simulink model "Fullmodelcontrol"  (R2020a)
settings: Solver=VariableStepAuto  StartTime=0.0  StopTime=10.0  RelTol=1e-3
values from neighbouring files (symbols this model uses):
  Ar = pi*D*D/4    (= 0.00465662571078)    [parameters.m]
  Cd = 0.23    [parameters.m]
  d = 0.081    [parameters.m]
  g = 9.81    [parameters.m]
  Ixx = 2.156e-3    (= 0.002156)    [parameters.m]
  l = 0.32    [parameters.m]
  m = 276.72e-3    (= 0.27672)    [parameters.m]
  rho = 1.225    [parameters.m]
  Thrust_timeC6 = (thrustprofileC6(:,1))'    [parameters.m]
  ThrustNtC6 = (thrustprofileC6(:,2))'    [parameters.m]
libraries: simulink x4, vrlib x2, dspsrcs4 x1
settings Model: Creator=sahil  LastModifiedBy=sahil

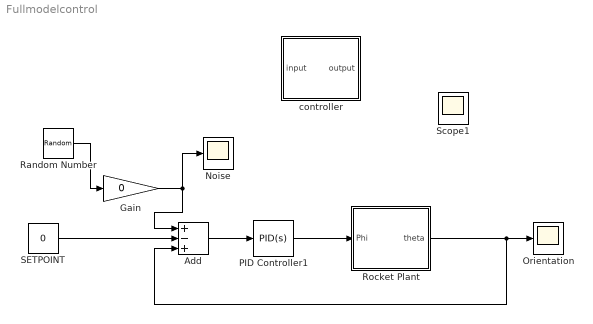
== system Fullmodelcontrol ==
  Add : Sum  Inputs=+-+
  Gain : Gain  Gain=0
  Noise : Scope
  Orientation : Scope
  PID Controller1 : simulink/Continuous/PID Controller  Controller=PID  Form=Parallel  TimeDomain=Continuous-time  UseExternalTs=off  SampleTime=-1  IntegratorMethod=Forward Euler  FilterMethod=Forward Euler  ControllerParametersSource=internal  P=0.142515145482664  I=0.0728938771028704  D=0.0532267076951464  UseFilter=on  N=36.46824066771  TunerSelectOption=Transfer Function Based (PID Tuner App)  InitialConditionSource=internal  InitialConditionForIntegrator=0  InitialConditionForFilter=0  DifferentiatorICPrevScaledInput=0  ExternalReset=none  TrackingMode=off  Kt=1  LimitOutput=on  UpperSaturationLimit=0.087  LowerSaturationLimit=-0.087  LinearizeAsGain=off  AntiWindupMode=none  Kb=1  POutMin=[]  POutMax=[]  IOutMin=[]  IOutMax=[]  DOutMin=[]  DOutMax=[]  NOutMin=[]  NOutMax=[]  SumOutMin=[]  SumOutMax=[]  SaturationOutMin=[]  SaturationOutMax=[]  PParamMin=[]  PParamMax=[]  IParamMin=[]  IParamMax=[]  DParamMin=[]  DParamMax=[]  NParamMin=[]  NParamMax=[]  KbParamMin=[]  KbParamMax=[]  KtParamMin=[]  KtParamMax=[]  KbOutMin=[]  KbOutMax=[]  KtOutMin=[]  KtOutMax=[]  IntegratorOutMin=[]  IntegratorOutMax=[]  FilterOutMin=[]  FilterOutMax=[]  SumI1OutMin=[]  SumI1OutMax=[]  SumI2OutMin=[]  SumI2OutMax=[]  SumI3OutMin=[]  SumI3OutMax=[]  SumI4OutMin=[]  SumI4OutMax=[]  SumDOutMin=[]  SumDOutMax=[]  DifferentiatorOutMin=[]  DifferentiatorOutMax=[]  FilterDiffOutCoefMin=[]  FilterDiffOutCoefMax=[]  ReciprocalOutMin=[]  ReciprocalOutMax=[]  SumDenOutMin=[]  SumDenOutMax=[]  SumNumOutMin=[]  SumNumOutMax=[]  DivideOutMin=[]  DivideOutMax=[]  UdiffTsProdOutMin=[]  UdiffTsProdOutMax=[]  NTsProdOutMin=[]  NTsProdOutMax=[]  UintegralTsProdOutMin=[]  UintegralTsProdOutMax=[]  UngainTsProdOutMin=[]  UngainTsProdOutMax=[]  IntegratorContinuousStateAttributes=''  IntegratorStateMustResolveToSignalObject=off  IntegratorRTWStateStorageClass=Auto  FilterContinuousStateAttributes=''  FilterStateMustResolveToSignalObject=off  FilterRTWStateStorageClass=Auto  ParallelPVariant=InternalParameters  IdealPVariant=Disabled  IVariant=InternalParameters  DVariant=InternalParameters  IntegratorVariant=Continuous  SatVariant=Enabled  AWVariant=Passthrough  PCopyVariant=Disabled  TRVariant=Disabled  FdbkBlocksVariant=Forward  IdealPFdbkVariant=Disabled  SatFdbkVariant=Disabled  DerivativeFilterVariant=ContFilter  NVariant=InternalParameters  NCopyVariant=Disabled  FilterICVariant=InternalICsFilter  IntegratorICVariant=InternalICs  ExternalResetVariant=Disabled  TRSumVariant=Passthrough  SumFdbkVariant=Disabled  SumVariant=Sum_PID  TsampFilterVariant=InternalTs  TsampNgainVariant=Passthrough  TsampIntegralVariant=Passthrough
  Random Number : RandomNumber  SampleTime=0.1
  Rocket Plant : Subsystem
  SETPOINT : Constant  Value=0
  Scope1 : Scope
  controller : Subsystem
  wires:
  Rocket Plant/1(theta) -> Add/3, Orientation/1
  PID Controller1/1 -> Rocket Plant/1(Phi)
  Random Number/1 -> Gain/1
  Gain/1 -> Add/1, Noise/1
  SETPOINT/1 -> Add/2
  Add/1 -> PID Controller1/1

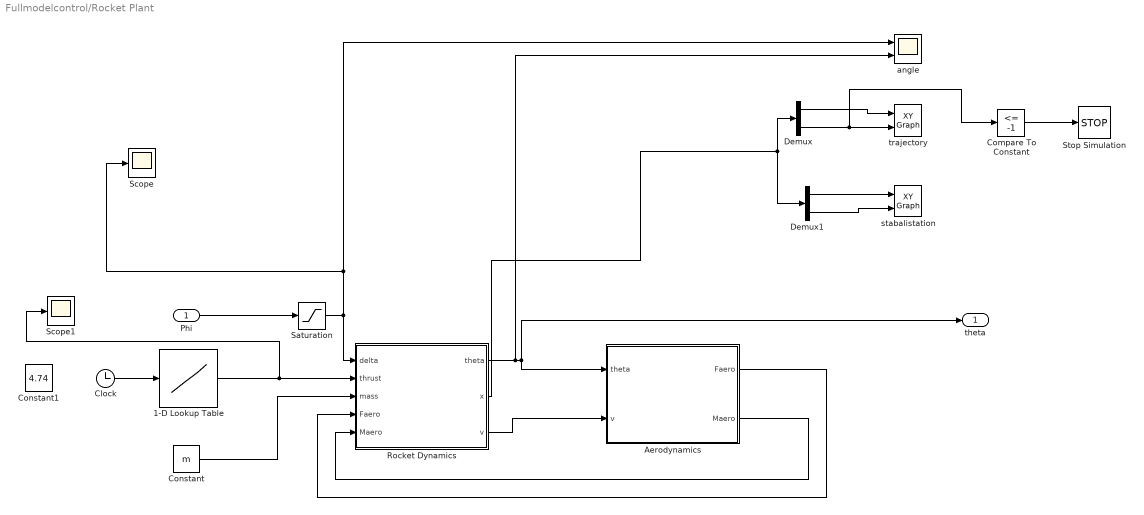
== system Fullmodelcontrol/Rocket Plant ==
  Phi : Inport
  1-D Lookup Table : Lookup_n-D  NumberOfTableDimensions=1  BreakpointsForDimension1=Thrust_timeC6  Table=ThrustNtC6  ExtrapMethod=Clip  InternalRulePriority=Speed  RndMeth=Simplest  InputSameDT=on
  Aerodynamics : Subsystem
  Clock : Clock
  Compare To Constant : simulink/Logic and Bit Operations/Compare To Constant  relop=<=  const=-1  OutDataTypeStr=boolean
  Constant : Constant  Value=m
  Constant1 : Constant  Value=4.74
  Demux : Demux  Outputs=2
  Demux1 : Demux  Outputs=2
  Rocket Dynamics : Subsystem
  Saturation : Saturate  UpperLimit=0.0873  LowerLimit=-0.0873
  Scope : Scope
  Scope1 : Scope
  Stop Simulation : Stop
  angle : Scope  NumInputPorts=2
  stabalistation : simulink/Sinks/XY Graph  xmin=-1  xmax=1  ymin=-5  ymax=50  st=-1
  trajectory : simulink/Sinks/XY Graph  xmin=-10  xmax=10  ymin=-5  ymax=30  st=-1
  theta : Outport
  wires:
  Rocket Dynamics/2(x) -> Demux1/1, Demux/1
  Demux1/2 -> stabalistation/2
  Aerodynamics/2(Maero) -> Rocket Dynamics/5(Maero)
  Clock/1 -> 1-D Lookup Table/1
  Demux1/1 -> stabalistation/1
  Saturation/1 -> Rocket Dynamics/1(delta), Scope/1, angle/1
  Rocket Dynamics/1(theta) -> angle/2, theta/1, Aerodynamics/1(theta)
  Demux/2 -> Compare To Constant/1, trajectory/2
  Aerodynamics/1(Faero) -> Rocket Dynamics/4(Faero)
  Constant/1 -> Rocket Dynamics/3(mass)
  Rocket Dynamics/3(v) -> Aerodynamics/2(v)
  Demux/1 -> trajectory/1
  Phi/1 -> Saturation/1
  1-D Lookup Table/1 -> Scope1/1, Rocket Dynamics/2(thrust)
  Compare To Constant/1 -> Stop Simulation/1

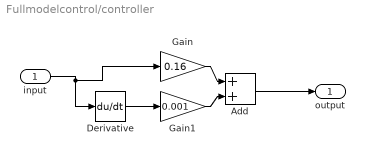
== system Fullmodelcontrol/controller ==
  input : Inport
  Add : Sum
  Derivative : Derivative
  Gain : Gain  Gain=0.16
  Gain1 : Gain  Gain=0.001
  output : Outport
  wires:
  Derivative/1 -> Gain1/1
  Gain/1 -> Add/1
  Gain1/1 -> Add/2
  input/1 -> Gain/1, Derivative/1
  Add/1 -> output/1

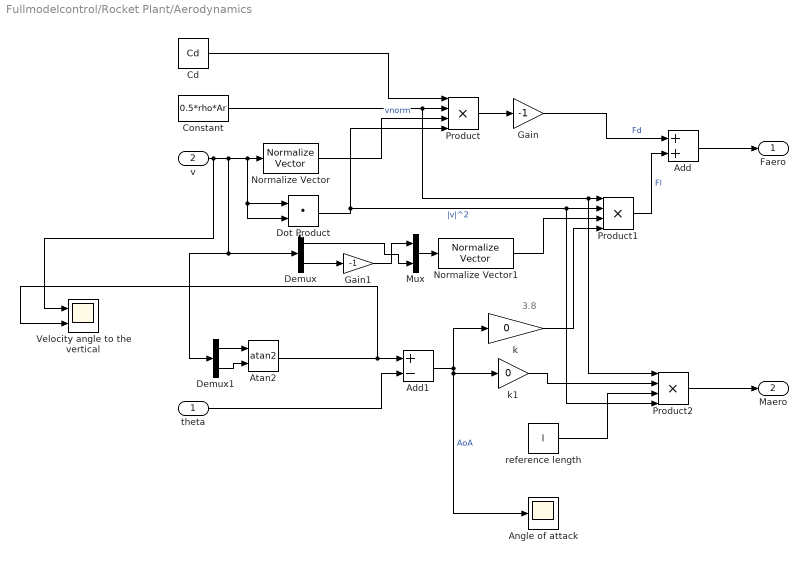
== system Fullmodelcontrol/Rocket Plant/Aerodynamics ==
  note: 3.8
  theta : Inport
  v : Inport  Port=2
  Add : Sum
  Add1 : Sum  Inputs=+-
  Angle of attack : Scope
  Atan2 : Trigonometry  Operator=atan2
  Cd : Constant  Value=Cd
  Constant : Constant  Value=0.5*rho*Ar
  Demux : Demux  Outputs=2
  Demux1 : Demux  Outputs=2
  Dot Product : DotProduct  InputSameDT=on  OutDataTypeStr=Inherit: Inherit via internal rule
  Gain : Gain  Gain=-1
  Gain1 : Gain  Gain=-1
  Mux : Mux  Inputs=2
  Normalize Vector : vrlib/Utilities/Normalize Vector  maxzero=0
  Normalize Vector1 : vrlib/Utilities/Normalize Vector  maxzero=0
  Product : Product  Inputs=4
  Product1 : Product  Inputs=4
  Product2 : Product  Inputs=4
  Velocity angle to the vertical : Scope  NumInputPorts=2
  k : Gain  Gain=0
  k1 : Gain  Gain=0
  reference length : Constant  Value=l
  Faero : Outport
  Maero : Outport  Port=2
  wires:
  v/1 -> Velocity angle to the vertical/1, Demux/1, Demux1/1, Dot Product/2, Dot Product/1, Normalize Vector/1
  Dot Product/1 -> Product/4, Product2/4, Product1/2  "|v|^2"
  Normalize Vector/1 -> Product/3  "vnorm"
  Constant/1 -> Product2/1, Product1/1, Product/2
  Product/1 -> Gain/1
  Demux/2 -> Gain1/1
  Gain1/1 -> Mux/1
  Demux/1 -> Mux/2
  Mux/1 -> Normalize Vector1/1
  Cd/1 -> Product/1
  Normalize Vector1/1 -> Product1/3
  Gain/1 -> Add/1  "Fd"
  Product1/1 -> Add/2  "Fl"
  Add/1 -> Faero/1
  Atan2/1 -> Velocity angle to the vertical/2, Add1/1
  theta/1 -> Add1/2
  Add1/1 -> k1/1, Angle of attack/1, k/1  "AoA"
  k/1 -> Product1/4
  reference length/1 -> Product2/3
  Product2/1 -> Maero/1
  Demux1/1 -> Atan2/1
  Demux1/2 -> Atan2/2
  k1/1 -> Product2/2

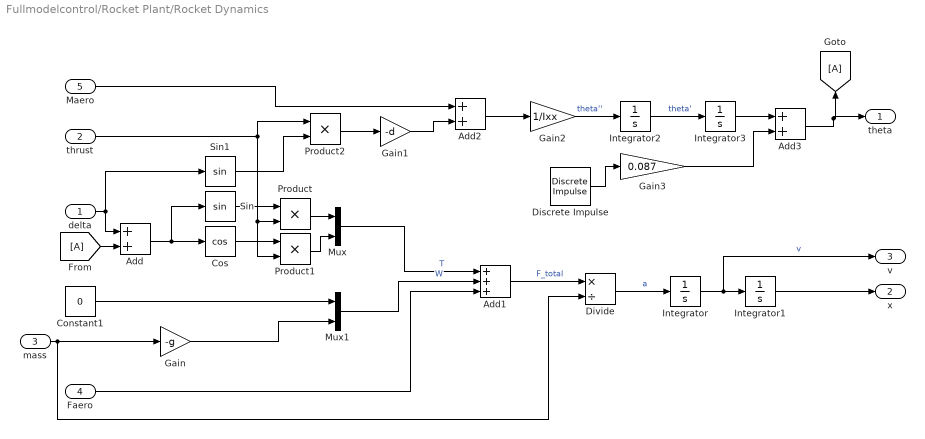
== system Fullmodelcontrol/Rocket Plant/Rocket Dynamics ==
  delta : Inport
  thrust : Inport  Port=2
  mass : Inport  Port=3
  Faero : Inport  Port=4
  Maero : Inport  Port=5
  Add : Sum
  Add1 : Sum  Inputs=+++
  Add2 : Sum
  Add3 : Sum
  Constant1 : Constant  Value=0
  Cos : Trigonometry  Operator=cos
  Discrete Impulse : dspsrcs4/Discrete  Impulse  Delay=3  SampleTime=0.1  FrameSample=1  OutputFrames=off  dataType=double  isSigned=on  wordLen=16  udDataType=sfix(16)  fracBitsMode=Best precision  numFracBits=15  OutDataTypeStr=double  LastOutDataTypeStr=double
  Divide : Product  Inputs=*/
  Gain : Gain  Gain=-g
  Gain1 : Gain  Gain=-d
  Gain2 : Gain  Gain=1/Ixx
  Gain3 : Gain  Gain=0.087
  Integrator{,1..3} (4 alike) : Integrator
  Mux : Mux  Inputs=2
  Mux1 : Mux  Inputs=2
  Product : Product
  Product1 : Product
  Product2 : Product
  Sin : Trigonometry
  Sin1 : Trigonometry
  theta : Outport
  x : Outport  Port=2
  v : Outport  Port=3
  wires:
  Add/1 -> Sin/1, Cos/1
  thrust/1 -> Product2/1, Product1/2, Product/2
  Sin/1 -> Product/1
  Cos/1 -> Product1/1
  Product/1 -> Mux/1
  Product1/1 -> Mux/2
  Mux/1 -> Add1/1  "T"
  mass/1 -> Divide/2, Gain/1
  Gain/1 -> Mux1/2
  Constant1/1 -> Mux1/1
  Mux1/1 -> Add1/2  "W"
  Faero/1 -> Add1/3
  Add1/1 -> Divide/1  "F_total"
  Divide/1 -> Integrator/1  "a"
  Integrator/1 -> v/1, Integrator1/1  "v"
  Integrator1/1 -> x/1
  delta/1 -> Sin1/1, Add/1
  [A] -> Add/2
  Sin1/1 -> Product2/2
  Product2/1 -> Gain1/1
  Gain1/1 -> Add2/2
  Maero/1 -> Add2/1
  Add2/1 -> Gain2/1
  Integrator2/1 -> Integrator3/1  "theta'"
  Gain2/1 -> Integrator2/1  "theta''"
  Integrator3/1 -> Add3/1
  Add3/1 -> [A], theta/1
  Discrete Impulse/1 -> Gain3/1
  Gain3/1 -> Add3/2
